simulink model "multipath"  (R2020b)
settings: Solver=VariableStepAuto  StartTime=0.0  StopTime=10.0  RelTol=1e-3
libraries: commrflib2 x2
settings Model: Creator=Yogapriya  LastModifiedBy=Yogapriya

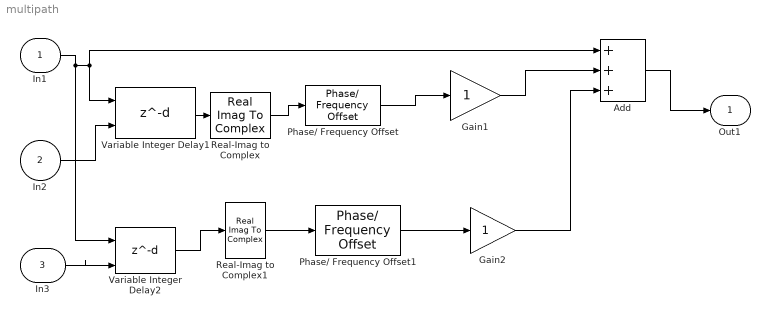
== system multipath ==
  In1 : Inport
  In2 : Inport  Port=2
  In3 : Inport  Port=3
  Add : Sum  Inputs=+++
  Gain1 : Gain
  Gain2 : Gain
  Phase/ Frequency Offset : commrflib2/Phase// Frequency Offset  phaseOffset=0  freqPort=off  freqOffset=0
  Phase/ Frequency Offset1 : commrflib2/Phase// Frequency Offset  phaseOffset=0  freqPort=off  freqOffset=0
  Real-Imag to Complex : RealImagToComplex  Input=Real
  Real-Imag to Complex1 : RealImagToComplex  Input=Real
  Variable Integer Delay1 : Delay  DelayLengthSource=Input port
      settings: InputPortMap=u0,p1
  Variable Integer Delay2 : Delay  DelayLengthSource=Input port
      settings: InputPortMap=u0,p1
  Out1 : Outport  SignalName=receiver
  wires:
  In1/1 -> Variable Integer Delay2/1, Variable Integer Delay1/1, Add/1
  In2/1 -> Variable Integer Delay1/2
  Phase/ Frequency Offset/1 -> Gain1/1
  Gain1/1 -> Add/2
  Add/1 -> Out1/1
  In3/1 -> Variable Integer Delay2/2
  Phase/ Frequency Offset1/1 -> Gain2/1
  Gain2/1 -> Add/3
  Variable Integer Delay2/1 -> Real-Imag to Complex1/1
  Real-Imag to Complex1/1 -> Phase/ Frequency Offset1/1
  Real-Imag to Complex/1 -> Phase/ Frequency Offset/1
  Variable Integer Delay1/1 -> Real-Imag to Complex/1
